simulink library "rayTraceBFGS_ul"  (R2018b)
settings: Solver=VariableStepAuto  StartTime=0.0  StopTime=10.0  RelTol=1e-3
values from neighbouring files (symbols this model uses):
  camDistances = []    [rayTraceBFGS_init.m]
  camFovAngs = []    [rayTraceBFGS_init.m]
  camIndxRefs = []    [rayTraceBFGS_init.m]
  camPosVecs = []    [rayTraceBFGS_init.m]
  camRotMats = []    [rayTraceBFGS_init.m]
  glassNormVecs = []    [rayTraceBFGS_init.m]
  glassThicknesses = []    [rayTraceBFGS_init.m]
  imageDims = []    [rayTraceBFGS_init.m]
settings Model: Creator=MAE-NCSUCORE  LastModifiedBy=M.Cobb

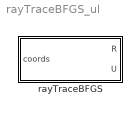
== system rayTraceBFGS_ul ==
  rayTraceBFGS : Subsystem  TreatAsAtomicUnit=on  mask{numOfCams=4, cam1PosVec=[0 0 1], cam1EulAng=[0 0 0], cam1Dist2Glass=1, cam1IdxRef=[1 1 1], cam1NormVec=[0 0 1], cam1GlassThick=1, cam1ImgDims=[1000 2000], cam1FoVAngs=[30 30], cam1NumDots=2, cam2PosVec=[0 0 1], cam2EulAng=[0 0 0], cam2Dist2Glass=1, cam2IdxRef=[1 1 1], cam2NormVec=[0 0 1], cam2GlassThick=1, cam2ImgDims=[1000 2000], cam2FoVAngs=[30 30], cam2NumDots=2, cam3PosVec=[0 0 1], cam3EulAng=[0 0 0], cam3Dist2Glass=1, cam3IdxRef=[1 1 1], cam3NormVec=[0 0 1], cam3GlassThick=1, cam3ImgDims=[1000 2000], cam3FoVAngs=[30 30], cam3NumDots=2, cam4PosVec=[0 0 1], cam4EulAng=[0 0 0], cam4Dist2Glass=1, cam4IdxRef=[1 1 1], cam4NormVec=[0 0 1], cam4GlassThick=1, cam4ImgDims=[1000 2000], cam4FoVAngs=[30 30], cam4NumDots=2, cam5PosVec=[0 0 1], cam5EulAng=[0 0 0], cam5Dist2Glass=1, cam5IdxRef=[1 1 1], cam5NormVec=[0 0 1], cam5GlassThick=1, cam5ImgDims=[1000 2000], cam5FoVAngs=[30 30], cam5NumDots=2}
      mask prompts: numOfCams "Number of Cameras"; cam1PosVec "Camera position vector (cm)"; cam1EulAng "Camera Euler angles (deg)"; cam1Dist2Glass "Distance 2 glass (cm)"; cam1IdxRef "Indices of refraction"; cam1NormVec "Glass out normal vector"; cam1GlassThick "Glass thickness (cm)"; cam1ImgDims "Image dimensions (px) [numRows numCols]"; cam1FoVAngs "Camera field of view angles (deg) [horiz vert]"; cam1NumDots "Number of dots tracked"; cam2PosVec "Camera position vector (cm)"; cam2EulAng "Camera Euler angles (deg)"; cam2Dist2Glass "Distance 2 glass (cm)"; cam2IdxRef "Indices of refraction"; cam2NormVec "Glass out normal vector"; cam2GlassThick "Glass thickness (cm)"; cam2ImgDims "Image dimensions (px) [numRows numCols]"; cam2FoVAngs "Camera field of view angles (deg) [horiz vert]"; cam2NumDots "Number of dots tracked"; cam3PosVec "Camera position vector (cm)"; cam3EulAng "Camera Euler angles (deg)"; cam3Dist2Glass "Distance 2 glass (cm)"; cam3IdxRef "Indices of refraction"; cam3NormVec "Glass out normal vector"; cam3GlassThick "Glass thickness (cm)"; cam3ImgDims "Image dimensions (px) [numRows numCols]"; cam3FoVAngs "Camera field of view angles (deg) [horiz vert]"; cam3NumDots "Number of dots tracked"; cam4PosVec "Camera position vector (cm)"; cam4EulAng "Camera Euler angles (deg)"; cam4Dist2Glass "Distance 2 glass (cm)"; cam4IdxRef "Indices of refraction"; cam4NormVec "Glass out normal vector"; cam4GlassThick "Glass thickness (cm)"; cam4ImgDims "Image dimensions (px) [numRows numCols]"; cam4FoVAngs "Camera field of view angles (deg) [horiz vert]"; cam4NumDots "Number of dots tracked"; cam5PosVec "Camera position vector (cm)"; cam5EulAng "Camera Euler angles (deg)"; cam5Dist2Glass "Distance 2 glass (cm)"; cam5IdxRef "Indices of refraction"; cam5NormVec "Glass out normal vector"; cam5GlassThick "Glass thickness (cm)"; cam5ImgDims "Image dimensions (px) [numRows numCols]"; cam5FoVAngs "Camera field of view angles (deg) [horiz vert]"; cam5NumDots "Number of dots tracked"
      mask init:
      | rayTraceBFGS_init
      mask Callback numOfCams: numOfCamsClbk
      mask DialogControl cam1Tab Prompt: Cam1
      mask DialogControl cam2Tab Prompt: Cam2
      mask DialogControl cam3Tab Prompt: Cam3
      mask DialogControl cam4Tab Prompt: Cam4
      mask DialogControl cam5Tab Prompt: Cam5

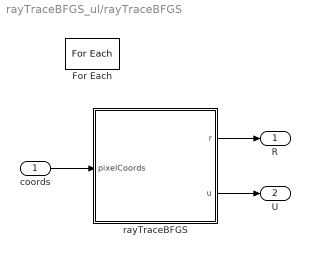
== system rayTraceBFGS_ul/rayTraceBFGS ==
  coords : Inport  Partition=on  PartitionDimension=1  PartitionWidth=1  PartitionOffset=0
  For Each : ForEach  DisableCoverage=on  IndexMode=One-based
  rayTraceBFGS : Subsystem  mask{camPosVec_cm=camPosVecs, grnd2CamRotMat=camRotMats, dist2Glass_cm=camDistances, indOfRefVec=camIndxRefs, glassOutNormalVec=glassNormVecs, glassThickness_cm=glassThicknesses, imageDimsVec_px=imageDims, camFOV_deg=camFovAngs}
      mask prompts: camPosVec_cm "Camera Position Vector, cm"; grnd2CamRotMat "Gnd 2 cam rotation matrix"; dist2Glass_cm "Distance to glass, cm"; indOfRefVec "Indices of refraction [air glass water]"; glassOutNormalVec "Glass outwards normal unit vector"; glassThickness_cm "Glass thickness, cm"; imageDimsVec_px "Image dimensions, px [rows cols]"; camFOV_deg "Camera field of view angles,deg  [horiz vert]"
      mask init:
      | % rayTrace_init
  R : Outport  ConcatenationDimension=1
  U : Outport  Port=2  ConcatenationDimension=1
  wires:
  coords/1 -> rayTraceBFGS/1(pixelCoords)
  rayTraceBFGS/1(r) -> R/1
  rayTraceBFGS/2(u) -> U/1

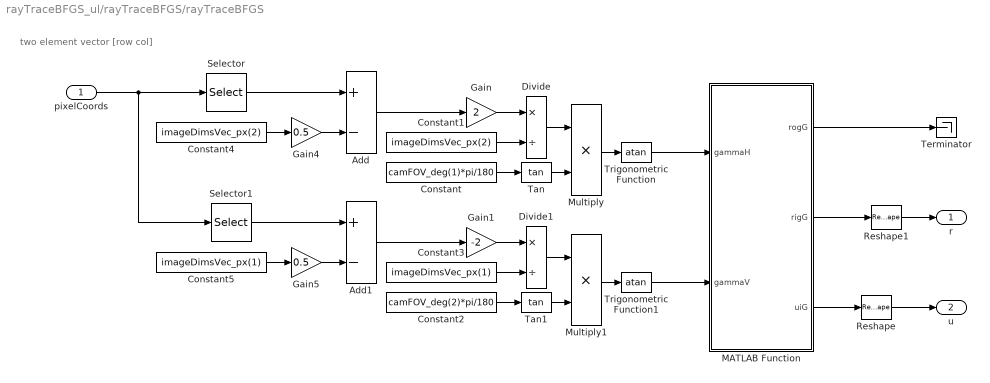
== system rayTraceBFGS_ul/rayTraceBFGS/rayTraceBFGS ==
  note: two element vector [row col]
  pixelCoords : Inport
  Add : Sum  Inputs=+-
  Add1 : Sum  Inputs=+-
  Constant : Constant  Value=camFOV_deg(1)*pi/180
  Constant1 : Constant  Value=imageDimsVec_px(2)
  Constant2 : Constant  Value=camFOV_deg(2)*pi/180
  Constant3 : Constant  Value=imageDimsVec_px(1)
  Constant4 : Constant  Value=imageDimsVec_px(2)
  Constant5 : Constant  Value=imageDimsVec_px(1)
  Divide : Product  Inputs=*/
  Divide1 : Product  Inputs=*/
  Gain : Gain  Gain=2
  Gain1 : Gain  Gain=-2
  Gain4 : Gain  Gain=0.5
  Gain5 : Gain  Gain=0.5
  MATLAB Function : MATLAB Function  TreatAsAtomicUnit=on
  Multiply : Product
  Multiply1 : Product
  Reshape : Reshape  OutputDimensionality=Column vector (2-D)
  Reshape1 : Reshape  OutputDimensionality=Column vector (2-D)
  Selector : Selector  InputPortWidth=2  IndexOptions=Index vector (dialog)  Indices=2  OutputSizes=1
  Selector1 : Selector  InputPortWidth=2  IndexOptions=Index vector (dialog)  Indices=1  OutputSizes=1
  Tan : Trigonometry  Operator=tan
  Tan1 : Trigonometry  Operator=tan
  Terminator : Terminator
  Trigonometric Function : Trigonometry  Operator=atan
  Trigonometric Function1 : Trigonometry  Operator=atan
  r : Outport
  u : Outport  Port=2
  wires:
  MATLAB Function/2(rigG) -> Reshape1/1
  MATLAB Function/3(uiG) -> Reshape/1
  MATLAB Function/1(rogG) -> Terminator/1
  Trigonometric Function/1 -> MATLAB Function/1(gammaH)
  Multiply/1 -> Trigonometric Function/1
  Tan/1 -> Multiply/2
  Constant/1 -> Tan/1
  Divide/1 -> Multiply/1
  Gain/1 -> Divide/1
  Constant1/1 -> Divide/2
  Gain1/1 -> Divide1/1
  Constant3/1 -> Divide1/2
  Constant2/1 -> Tan1/1
  Trigonometric Function1/1 -> MATLAB Function/2(gammaV)
  Multiply1/1 -> Trigonometric Function1/1
  Tan1/1 -> Multiply1/2
  Divide1/1 -> Multiply1/1
  pixelCoords/1 -> Selector1/1, Selector/1
  Add/1 -> Gain/1
  Constant4/1 -> Gain4/1
  Gain4/1 -> Add/2
  Constant5/1 -> Gain5/1
  Gain5/1 -> Add1/2
  Add1/1 -> Gain1/1
  Selector/1 -> Add/1
  Selector1/1 -> Add1/1
  Reshape1/1 -> r/1
  Reshape/1 -> u/1

== matlab function rayTraceBFGS_ul/rayTraceBFGS/rayTraceBFGS/MATLAB Function ==
  data: rogG output; rigG output; gammaH input; gammaV input; uiG output; camPosVec_cm parameter; grnd2CamRotMat parameter; dist2Glass_cm parameter; indOfRefVec parameter; glassOutNormalVec parameter; glassThickness_cm parameter
function [rogG,rigG,uiG] = ...
    rayTrace(gammaH,gammaV,camPosVec_cm,grnd2CamRotMat,dist2Glass_cm,...
    indOfRefVec,glassOutNormalVec,glassThickness_cm)

[rogG,rigG,uiG] = ...
    rayTraceBFGS(camPosVec_cm,grnd2CamRotMat,dist2Glass_cm,gammaH,gammaV,...
    indOfRefVec,glassOutNormalVec,glassThickness_cm);
